simulink model "vehicle_model"  (R2017b)
settings: Solver=VariableStepAuto  StartTime=0.0  StopTime=100  RelTol=1e-3
values from neighbouring files (symbols this model uses):
  d = 0.10    (= 0.1)    [main.m]
  R = 0.056/2    (= 0.028)    [main.m]
undefined symbols (not defined in the file or in its folder): lkk, lP12, lP1P2, q1, q2, rkk, rP12, rP1P2
libraries: simulink x4, dspstat3 x2
settings Model: Creator=hoh  LastModifiedBy=hoh

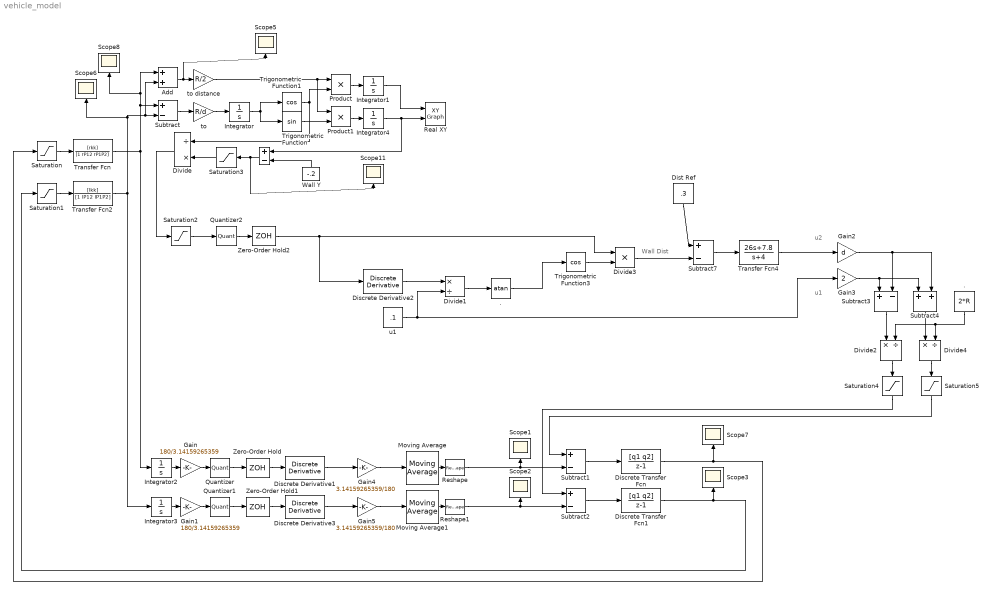
== system vehicle_model ==
  note: Wall Dist
  note: u2
  note: u1
  "   " : Sum  Inputs=+-
  . : Trigonometry  Operator=atan
  ". " : Constant  Value=2*R
  Add : Sum
  Discrete Transfer Fcn : DiscreteTransferFcn  Numerator=[q1 q2]  Denominator=[1 -1]
  Discrete Transfer Fcn1 : DiscreteTransferFcn  Numerator=[q1 q2]  Denominator=[1 -1]
  Discrete Derivative1 : simulink/Discrete/Discrete Derivative  gainval=1  ICPrevScaledInput=0  OutMin=[]  OutMax=[]  OutDataType=fixdt(1, 16)  OutScaling=2^-10  DoSatur=off
  Discrete Derivative2 : simulink/Discrete/Discrete Derivative  gainval=1  ICPrevScaledInput=0  OutMin=[]  OutMax=[]  OutDataType=fixdt(1, 16)  OutScaling=2^-10  DoSatur=off
  Discrete Derivative3 : simulink/Discrete/Discrete Derivative  gainval=1  ICPrevScaledInput=0  OutMin=[]  OutMax=[]  OutDataType=fixdt(1, 16)  OutScaling=2^-10  DoSatur=off
  Dist Ref : Constant  Value=.3
  Divide : Product  Inputs=/*
  Divide1 : Product  Inputs=*/
  Divide2 : Product  Inputs=*/
  Divide3 : Product  Inputs=**
  Divide4 : Product  Inputs=*/
  Gain : Gain  Gain=180/3.14159265359
  Gain1 : Gain  Gain=180/3.14159265359
  Gain2 : Gain  Gain=d
  Gain3 : Gain  Gain=2
  Gain4 : Gain  Gain=3.14159265359/180
  Gain5 : Gain  Gain=3.14159265359/180
  Integrator{,1..4} (5 alike) : Integrator
  Moving Average : dspstat3/Moving Average  Method=Exponential weighting  SpecifyWindowLength=on  WindowLength=3  ForgettingFactor=.6  SimulateUsing=Code generation
  Moving Average1 : dspstat3/Moving Average  Method=Sliding window  SpecifyWindowLength=on  WindowLength=4  ForgettingFactor=0.6  SimulateUsing=Code generation
  Product : Product
  Product1 : Product
  Quantizer : Quantizer  QuantizationInterval=1
  Quantizer1 : Quantizer  QuantizationInterval=1
  Quantizer2 : Quantizer  QuantizationInterval=.01
  Real XY : simulink/Sinks/XY Graph  xmin=0  xmax=5  ymin=-5  ymax=1  st=-1
  Reshape : Reshape
  Reshape1 : Reshape
  Saturation : Saturate  UpperLimit=100  LowerLimit=0
  Saturation1 : Saturate  UpperLimit=100  LowerLimit=0
  Saturation2 : Saturate  UpperLimit=1.5  LowerLimit=.02
  Saturation3 : Saturate  UpperLimit=100  LowerLimit=0
  Saturation4 : Saturate  UpperLimit=12  LowerLimit=0
  Saturation5 : Saturate  UpperLimit=12  LowerLimit=0
  Scope{1..3,5..8,11} (8 alike) : Scope
  Subtract{,1..3,7} (5 alike) : Sum  Inputs=+-
  Subtract4 : Sum
  Transfer Fcn : TransferFcn  Numerator=[rkk]  Denominator=[1 rP12 rP1P2]
  Transfer Fcn2 : TransferFcn  Numerator=[lkk]  Denominator=[1 lP12 lP1P2]
  Transfer Fcn4 : TransferFcn  Numerator=[26 7.8]  Denominator=[1 4]
  Trigonometric Function : Trigonometry
  Trigonometric Function1 : Trigonometry  Operator=cos
  Trigonometric Function3 : Trigonometry  Operator=cos
  Wall Y : Constant  Value=-.2
  Zero-Order Hold : ZeroOrderHold  SampleTime=0.005
  Zero-Order Hold1 : ZeroOrderHold  SampleTime=0.005
  Zero-Order Hold2 : ZeroOrderHold  SampleTime=0.2
  "to " : Gain  Gain=R/d
  to distance : Gain  Gain=R/2
  u1 : Constant  Value=.1
  wires:
  Subtract/1 -> "to "/1
  Integrator/1 -> Trigonometric Function/1, Trigonometric Function1/1
  to distance/1 -> Product1/1, Product/1
  Product/1 -> Integrator1/1
  Integrator1/1 -> Real XY/1
  Product1/1 -> Integrator4/1
  Add/1 -> Scope5/1, to distance/1
  "to "/1 -> Integrator/1
  Integrator2/1 -> Gain/1
  Quantizer/1 -> Zero-Order Hold/1
  Quantizer1/1 -> Zero-Order Hold1/1
  Gain1/1 -> Quantizer1/1
  Integrator3/1 -> Gain1/1
  Trigonometric Function/1 -> Product1/2
  Saturation1/1 -> Transfer Fcn2/1
  Saturation/1 -> Transfer Fcn/1
  Quantizer2/1 -> Zero-Order Hold2/1
  Divide/1 -> Saturation2/1
  Saturation2/1 -> Quantizer2/1
  Integrator4/1 -> "   "/1, Real XY/2
  Trigonometric Function1/1 -> Product/2, Divide/1
  Transfer Fcn2/1 -> Integrator3/1, Scope6/1, Subtract/2, Add/2
  Zero-Order Hold/1 -> Discrete Derivative1/1
  Zero-Order Hold1/1 -> Discrete Derivative3/1
  Wall Y/1 -> "   "/2
  "   "/1 -> Scope11/1, Saturation3/1
  Saturation3/1 -> Divide/2
  Discrete Derivative1/1 -> Gain4/1
  Moving Average/1 -> Reshape/1
  Discrete Derivative3/1 -> Gain5/1
  Moving Average1/1 -> Reshape1/1
  Gain4/1 -> Moving Average/1
  Gain5/1 -> Moving Average1/1
  Gain/1 -> Quantizer/1
  Subtract1/1 -> Discrete Transfer Fcn/1
  Subtract2/1 -> Discrete Transfer Fcn1/1
  Discrete Transfer Fcn/1 -> Saturation/1, Scope7/1
  Discrete Transfer Fcn1/1 -> Saturation1/1, Scope3/1
  Reshape/1 -> Subtract1/2, Scope1/1
  Reshape1/1 -> Subtract2/2, Scope2/1
  Transfer Fcn/1 -> Scope8/1, Add/1, Subtract/1, Integrator2/1
  Discrete Derivative2/1 -> Divide1/1
  Divide1/1 -> ./1
  Saturation4/1 -> Subtract2/1
  Saturation5/1 -> Subtract1/1
  Dist Ref/1 -> Subtract7/1
  Subtract7/1 -> Transfer Fcn4/1
  Trigonometric Function3/1 -> Divide3/2
  Divide3/1 -> Subtract7/2
  ./1 -> Trigonometric Function3/1
  Zero-Order Hold2/1 -> Divide3/1, Discrete Derivative2/1
  u1/1 -> Gain3/1, Divide1/2
  Transfer Fcn4/1 -> Gain2/1
  Gain3/1 -> Subtract4/1, Subtract3/1
  Gain2/1 -> Subtract4/2, Subtract3/2
  ". "/1 -> Divide2/2, Divide4/2
  Subtract3/1 -> Divide2/1
  Subtract4/1 -> Divide4/1
  Divide2/1 -> Saturation4/1
  Divide4/1 -> Saturation5/1
